simulink model "VariousSpeed2018_14dof_ypredictor_sc"  (R2017a)
settings: Solver=ode4  StartTime=0.0  StopTime=70  FixedStep=dt  RelTol=1e-3
values from neighbouring files (symbols this model uses):
  g_motor_eff = 1    [VESIM_init.m]
  gr_motor = 0    [VESIM_init.m]
undefined symbols (not defined in the file or in its folder): A_mc, brake_Pw, brake_V, C_q, diff_efficiency, diff_wRatio, dt, engine_inertia, error_lookuptable, F_cf, F_cs, fmin_mg, fmin_mg_na, J_cal, K_vb, Kp_rpm, mdot_fuel, model_lookuptable, no_cyl, P_0, P_gain, rpm0_c, rpm2rads, rpm_e, rpm_hi_idle, rpm_idle, rpm_max_c, rpm_rated, Standard_Devices, Ti_rpm, torque_engine, trq_scale, Tt_rpm, UDP_Protocol, vdes, Xobs, Yobs
libraries: simulink x10, vrlib x3, sldrtlib x3, SimulinkExecutionControl x1
(part 1 of 2)
settings Model: SimulationMode=accelerator  Creator=wenyifan  LastModifiedBy=Chen Li
settings SolverCC: AlgebraicLoopSolver=LineSearch
settings DataIOCC: LimitDataPoints=on  SaveFormat=Array
settings OptimizationCC: BlockReduction=off  BooleanDataType=off  LifeSpan=inf
settings DebuggingCC: SaveWithParameterizedLinksMsg=none  UnderspecifiedInitializationDetection=Classic  MergeDetectMultiDrivingBlocksExec=none  SignalResolutionControl=TryResolveAllWithWarning  AllowSymbolicDim=off  SFUnexpectedBacktrackingDiag=warning  SFNoUnconditionalDefaultTransitionDiag=warning  SFExecutionAtInitializationDiag=none
settings HardwareCC: TargetBitPerLong=64  TargetBitPerPointer=64  TargetIntDivRoundTo=Zero  TargetEndianess=LittleEndian  TargetWordSize=64  TargetHWDeviceType=Intel->x86-64
settings ModelReferenceCC: PropagateSignalLabelsOutOfModel=off
settings SFSimCC: MATLABDynamicMemAlloc=off
settings RTWCC: SystemTargetFile=sldrtert.tlc  TemplateMakefile=sldrtert.tmf  Description=Simulink Desktop Real-Time (ERT)  RTWCompilerOptimization=on
settings CodeAppCC: MaxIdLength=95
settings SimulinkDesktopRealTimeERTCC: TargetFcnLib=ansi_tfl_table_tmw.mat  TargetLibSuffix=_sldrt.lib  TargetPreCompLibLocation=E:\Matlab_2019a\toolbox\sldrt\lib\win64  GenFloatMathFcnCalls=NOT IN USE  TargetLangStandard=C89/C90 (ANSI)  CodeReplacementLibrary=None  UtilityFuncGeneration=Auto  MultiwordTypeDef=System defined  MultiwordLength=2048  GenerateFullHeader=on  InferredTypesCompatibility=off  GenerateSampleERTMain=off  GenerateTestInterfaces=off  ModelReferenceCompliant=on  ParMdlRefBuildCompliant=off  CompOptLevelCompliant=on  ConcurrentExecutionCompliant=off  IncludeMdlTerminateFcn=on  GeneratePreprocessorConditionals=Use local settings  CombineOutputUpdateFcns=off  CombineSignalStateStructs=off  SuppressErrorStatus=off  IncludeFileDelimiter=Auto  ERTCustomFileBanners=off  SupportAbsoluteTime=on  LogVarNameModifier=rt_  MatFileLogging=off  MultiInstanceERTCode=off  CodeInterfacePackaging=Nonreusable function  SupportNonFinite=on  SupportComplex=on  PurelyIntegerCode=off  SupportContinuousTime=on  SupportNonInlinedSFcns=on  RemoveDisableFunc=off  RemoveResetFunc=on  SupportVariableSizeSignals=off  ParenthesesLevel=Nominal  CastingMode=Nominal  MATLABClassNameForMDSCustomization=Simulink.SoftwareTarget.TargetSpecificTriggerConfigurationBase  ModelStepFunctionPrototypeControlCompliant=off  CPPClassGenCompliant=off  AutosarCompliant=off  MDXCompliant=off  GRTInterface=off  GenerateAllocFcn=off  UseToolchainInfoCompliant=off  GenerateSharedConstants=on  CoderGroups=[]  AccessMethods=[]  LookupTableObjectStructAxisOrder=1,2,3,4,...  GenerateASAP2=off  InlinedParameterPlacement=Hierarchical  TargetOS=BareBoardExample  MultiInstanceErrorCode=Error  RootIOFormat=Individual arguments  RTWCAPISignals=off  RTWCAPIParams=off  RTWCAPIStates=off  RTWCAPIRootIO=off  ERTSrcFileBannerTemplate=ert_code_template.cgt  ERTHdrFileBannerTemplate=ert_code_template.cgt  ERTDataSrcFileTemplate=ert_code_template.cgt  ERTDataHdrFileTemplate=ert_code_template.cgt  ERTCustomFileTemplate=example_file_process.tlc  EnableDataOwnership=off  SignalDisplayLevel=10  ParamTuneLevel=10  GlobalDataDefinition=Auto  DataDefinitionFile=global.c  GlobalDataReference=Auto  ERTFilePackagingFormat=Modular  DataReferenceFile=global.h  PreserveExpressionOrder=off  PreserveIfCondition=off  ConvertIfToSwitch=off  PreserveExternInFcnDecls=on  SuppressUnreachableDefaultCases=off  EnableSignedLeftShifts=on  EnableSignedRightShifts=on  IndentStyle=K&R  IndentSize=2  EnableUserReplacementTypes=off  MaxIdInt32=MAX_int32_T  MinIdInt32=MIN_int32_T  MaxIdUint32=MAX_uint32_T  MaxIdInt16=MAX_int16_T  MinIdInt16=MIN_int16_T  MaxIdUint16=MAX_uint16_T  MaxIdInt8=MAX_int8_T  MinIdInt8=MIN_int8_T  MaxIdUint8=MAX_uint8_T  BooleanTrueId=true  BooleanFalseId=false  MemSecPackage=--- None ---  MemSecDataConstants=Default  MemSecDataIO=Default  MemSecDataInternal=Default  MemSecDataParameters=Default  MemSecFuncInitTerm=Default  MemSecFuncExecute=Default  MemSecFuncSharedUtil=Default  GroupConstants=Default  GroupRootInputs=Default  GroupRootOutputs=Default  GroupInternal=Default  GroupParameters=Default  GroupDataTransfer=Default  GroupInstanceSpecificParameters=Default  GroupModelData=Default  CCListing=off  RebuildAll=off  ExtMode=on  ExtModeTransport=0  ExtModeStaticAlloc=off  ExtModeStaticAllocSize=1000000  ExtModeTesting=off  ExtModeMexFile=sldrtext  ExtModeIntrfLevel=Level1
settings ConfigComp: CovMetricSettings=dw  CovHtmlReporting=on  CovSaveCumulativeToWorkspaceVar=on  CovSaveSingleToWorkspaceVar=on  CovExternalEMLEnable=off  CovSFcnEnable=off

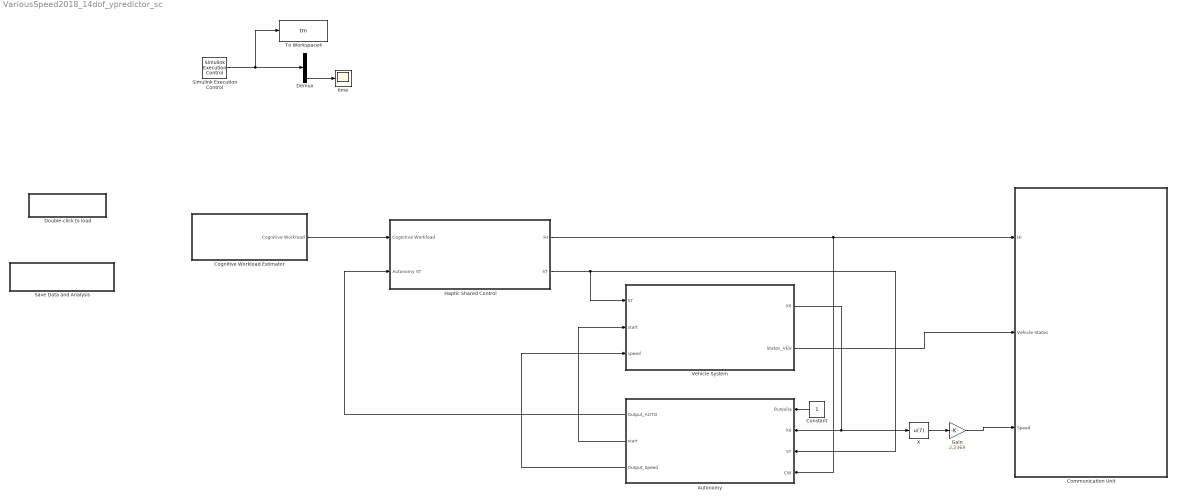
== system VariousSpeed2018_14dof_ypredictor_sc ==
  Autonomy : Subsystem
  Cognitive Workload Estimator : Subsystem
  Communication Unit : Subsystem
  Constant : Constant
  Demux : Demux  Outputs=3
  Double-click to load : Subsystem
      settings: OpenFcn=|
      | close all;
      | clear all;
      | clc;
      | 
      | env_init;
      | addpath(genpath(pwd))
      | 
      | 
      | VESIM_init;
      | VEHICLE14DoF_init;
      mask Help: This block runs/ndes_init.m file in the main directory
      mask Display: disp('Load Parameters')
  Gain : Gain  Gain=2.2369
  Haptic Shared Control : Subsystem
  Save Data and Analysis : Subsystem
      settings: OpenFcn=post_processing_analysis_pred_sc;
      mask Help: This block runs/ndes_init.m file in the main directory
      mask Display: disp('Save Data and Analysis')
  Simulink Execution Control : SimulinkExecutionControl/Simulink Execution Control  proc_pri=ABOVE_NORMAL_PRIORITY_CLASS  thread_pri=THREAD_PRIORITY_NORMAL  rt_sim=on  factor=1  ovrrun=Continue execution  Ts=dt
  To Workspace4 : ToWorkspace  VariableName=tm  SampleTime=-1
  Vehicle System : Subsystem
  X : Fcn  Expr=u(7)
  time : Scope
  wires:
  Simulink Execution Control/1 -> To Workspace4/1, Demux/1
  Vehicle System/1(X0) -> Autonomy/2(X0), X/1
  Constant/1 -> Autonomy/1(RunJulia)
  Haptic Shared Control/1(HI) -> Autonomy/4(CW), Communication Unit/1(HI)
  Demux/3 -> time/1
  Autonomy/3(Output_Speed) -> Vehicle System/3(speed)
  Gain/1 -> Communication Unit/3(Speed)
  Vehicle System/2(States_VEH) -> Communication Unit/2(Vehicle States)
  Autonomy/2(start) -> Vehicle System/2(start)
  X/1 -> Gain/1
  Autonomy/1(Output_AUTO) -> Haptic Shared Control/2(Autonomy ST)
  Cognitive Workload Estimator/1(Cognitive Workload) -> Haptic Shared Control/1(Cognitive Workload)
  Haptic Shared Control/2(ST) -> Vehicle System/1(ST), Autonomy/3(ST)

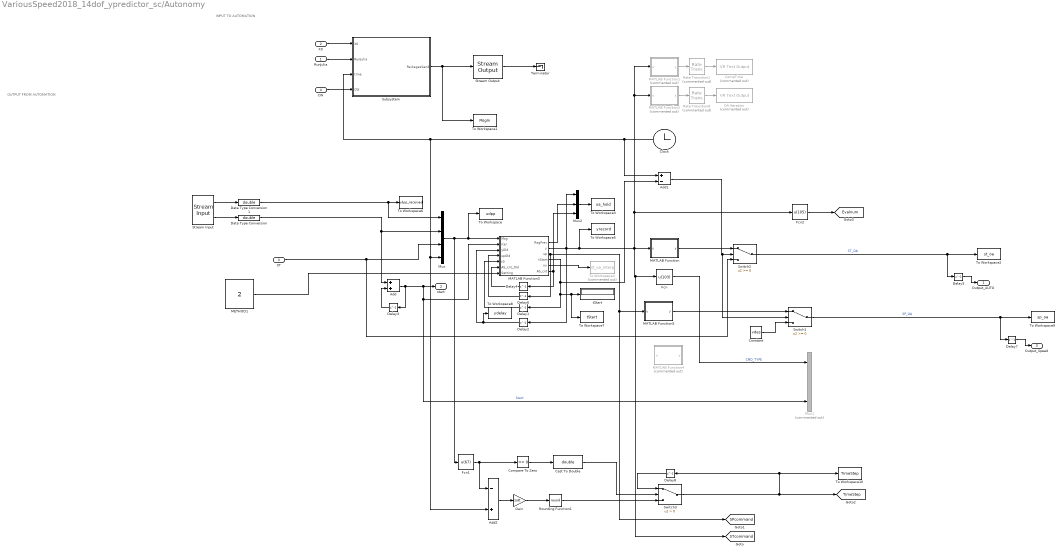
== system VariousSpeed2018_14dof_ypredictor_sc/Autonomy ==
  note: OUTPUT FROM AUTOMATION
  note: INPUT TO AUTOMATION
  RunJulia : Inport
  X0 : Inport  Port=2
  ST : Inport  Port=3
  CW : Inport  Port=4
  Add : Sum
  Add1 : Sum  Inputs=+-
  Add2 : Sum  Inputs=-+
  Cast To Double : DataTypeConversion  OutDataTypeStr=double
  Clock : Clock
      settings: Decimation=100
  CompTime : vrlib/VR Text Output  Commented=on  Ts=-1  ForceViewerOpen=off
      settings: SourceProductName=Simulink 3D Animation  SourceProductBaseCode=VR
  Compare To Zero : simulink/Logic and Bit Operations/Compare To Zero  relop===  OutDataTypeStr=boolean
  Constant : Constant  Value=vdes
  Data Type Conversion : DataTypeConversion  OutDataTypeStr=double
  Data Type Conversion1 : DataTypeConversion  OutDataTypeStr=double
  Delay{1,3..5,7..8} (6 alike) : Delay  DelayLength=1  InitialCondition=0  SampleTime=dt
  Delay2 : Delay  DelayLength=1  InitialCondition=zeros(110,1)  SampleTime=dt
  Delay6 : Delay  DelayLength=1  InitialCondition=zeros(110,1)  SampleTime=dt
  Fcn : Fcn  Expr=u(103)
  Fcn1 : Fcn  Expr=u(67)
  Fcn2 : Fcn  Expr=u(105)
  Gain : Gain  Gain=1/dt
  MATLAB Function : MATLAB Function  TreatAsAtomicUnit=on
  MATLAB Function1 : MATLAB Function  Commented=on  TreatAsAtomicUnit=on
  MATLAB Function2 : MATLAB Function  Commented=on  TreatAsAtomicUnit=on
  MATLAB Function3 : MATLAB Function  TreatAsAtomicUnit=on
  MATLAB Function4 : MATLAB Function  Commented=on  TreatAsAtomicUnit=on
  MATLAB Function5 : MATLAB Function  TreatAsAtomicUnit=on
  METHOD1 : Constant  Value=2
  Mux : Mux
  Mux1 : Mux  Commented=on  Inputs=3
  Mux2 : Mux  Inputs=3
  OA Iteration : vrlib/VR Text Output  Commented=on  Ts=-1  ForceViewerOpen=off
      settings: SourceProductName=Simulink 3D Animation  SourceProductBaseCode=VR
  Rate Transition1 : RateTransition  Commented=on
  Rate Transition8 : RateTransition  Commented=on
  Rounding Function1 : Rounding  Operator=round
  Stream Input : sldrtlib/Stream Input  SampleTime=0.01  MaxMissedTicks=Inf  ShowMissedTicks=off  YieldWhenWaiting=off  DrvName=Standard_Devices/UDP_Protocol  DrvAddress=36881  DrvOptions=[0 12000 51 53 46 51 46 57 57 46 49 57 53 0 0 0 0 0 0 0 0 0 0 0 0 0 0 0 0 0 0 0 0 0 0 0 0 0 0 0 0 0 0 0 0 0 0 0 0 0 0 0 0 0 0 0 0 0 0 0 0 0 0 0 0 0 0 0 0 0 0 0 0 0 0 0 0 0 0 0 0 0 0 0 0 0 0 0 0 0 0 0 0 0 0 0 0 0 0 0 0 0 0 0 0 0 0 0 0 0 0 0 0 0 0 0 0 0 0 0 0 0 0 0 0 0 0 0 0 0 0 0 0 0 0 0 0 0 0 0 0 0 0 0 0 0 0 0 0 0 0 0 0 0 0 0 0 0 0 0 0 0 0 0 0 0 0 0 0 0 0 0 0 0 0 0 0 0 0 0 0 0 0 0 0 0 0 0 0 0 0 0 0 0 0 0 0 0 0 0 0 0 0 0 0 0 0 0 0 0 0 0 0 0 0 0 0 0 0 0 0 0 0 0 0 0 0 0 0 0 0 0 0 0 0 0 0 0 0 0 0 0 0 0 0 0 0 0 0 0 0 0 0 0 0 0]  DataTypes={'68*double'}  FormatString='%f,%f,%f,%f,%f,%f,%f,%f,%f,%f,%f,%f,%f,%f,%f,%f,%f,%f,%f,%f,%f,%f,%f,%f,%f,%f,%f,%f,%f,%f,%f,%f,%f,%f,%f,%f,%f,%f,%f,%f,%f,%f,%f,%f,%f,%f,%f,%f,%f,%f,%f,%f,%f,%f,%f,%f,%f,%f,%f,%f,%f,%f,%f,%f,%f,%f,%f,%f'  Terminator={ '\r', '\n' }  ShowReady=on  ShowError=off
      settings: AttributesFormatString=UDP Protocol [36881]  SourceProductName=Simulink Desktop Real-Time  SourceProductBaseCode=WT
  Stream Output : sldrtlib/Stream Output  SampleTime=0.01  MaxMissedTicks=Inf  ShowMissedTicks=on  YieldWhenWaiting=off  DrvName=Standard_Devices/UDP_Protocol  DrvAddress=36864  DrvOptions=[0 36880 51 53 46 51 46 57 57 46 49 57 53 0 0 0 0 0 0 0 0 0 0 0 0 0 0 0 0 0 0 0 0 0 0 0 0 0 0 0 0 0 0 0 0 0 0 0 0 0 0 0 0 0 0 0 0 0 0 0 0 0 0 0 0 0 0 0 0 0 0 0 0 0 0 0 0 0 0 0 0 0 0 0 0 0 0 0 0 0 0 0 0 0 0 0 0 0 0 0 0 0 0 0 0 0 0 0 0 0 0 0 0 0 0 0 0 0 0 0 0 0 0 0 0 0 0 0 0 0 0 0 0 0 0 0 0 0 0 0 0 0 0 0 0 0 0 0 0 0 0 0 0 0 0 0 0 0 0 0 0 0 0 0 0 0 0 0 0 0 0 0 0 0 0 0 0 0 0 0 0 0 0 0 0 0 0 0 0 0 0 0 0 0 0 0 0 0 0 0 0 0 0 0 0 0 0 0 0 0 0 0 0 0 0 0 0 0 0 0 0 0 0 0 0 0 0 0 0 0 0 0 0 0 0 0 0 0 0 0 0 0 0 0 0 0 0 0 0 0 0 0 0 0 0 0]  PortSizes=[23]  FormatString='%f %f %f %f %f %f %f %f %f %f %f %f %f %f %f %f %f %f %f %f %f %f %f \n'  ShowReady=off  ShowError=off  InitialValue=[]  FinalValue=[]
      settings: AttributesFormatString=UDP Protocol [36864]  SourceProductName=Simulink Desktop Real-Time  SourceProductBaseCode=WT
  Subsystem : Subsystem
  Switch1 : Switch
  Switch2 : Switch
  Switch3 : Switch  Criteria=u2 > Threshold
  Terminator : Terminator
  To Workspace : ToWorkspace  VariableName=udpp  SampleTime=-1
      settings: Save2DSignal=2-D array (concatenate along first dimension)
  To Workspace1 : ToWorkspace  VariableName=MsgIn  SampleTime=-1
  To Workspace10 : ToWorkspace  VariableName=TimeStep  SampleTime=-1
  To Workspace2 : ToWorkspace  VariableName=st_oa  SampleTime=-1
  To Workspace3 : ToWorkspace  VariableName=oa_hold  SampleTime=-1
  To Workspace4 : ToWorkspace  Commented=on  VariableName=st_oa_interp  SampleTime=-1
  To Workspace5 : ToWorkspace  VariableName=yrecord  SampleTime=-1
      settings: Save2DSignal=2-D array (concatenate along first dimension)
  To Workspace6 : ToWorkspace  VariableName=udpp_received  SampleTime=-1
      settings: Save2DSignal=2-D array (concatenate along first dimension)
  To Workspace7 : ToWorkspace  VariableName=tStart  SampleTime=-1
  To Workspace8 : ToWorkspace  VariableName=ydelay  SampleTime=-1
      settings: Save2DSignal=2-D array (concatenate along first dimension)
  To Workspace9 : ToWorkspace  VariableName=sp_oa  SampleTime=-1
  tStart : Display
  Output_AUTO : Outport
  start : Outport  Port=2
  Output_Speed : Outport  Port=3
  tag scope: Evalnum=global, SPcommand=global, STcommand=global, TimeStep=global
  wires:
  Data Type Conversion1/1 -> Mux/1, To Workspace6/1
  MATLAB Function3/5(uu) -> To Workspace4/1
  MATLAB Function/1(y) -> Switch2/1
  Add1/1 -> Switch1/2, Switch2/2
  Add/1 -> Delay3/1, Mux1/3, MATLAB Function3/2(iter), start/1  "Start"
  Subsystem/1(PackagesSend) -> Stream Output/1, To Workspace1/1
  Rate Transition8/1 -> OA Iteration/1
  MATLAB Function3/6(AS_cnt) -> Mux2/3, Delay4/1
  Fcn/1 -> Mux1/1  "CMD_TYPE"
  MATLAB Function2/1(y) -> Rate Transition8/1
  Rate Transition1/1 -> CompTime/1
  MATLAB Function3/4(tStart) -> Add1/2, Delay1/1, To Workspace7/1, tStart/1
  Delay4/1 -> MATLAB Function3/6(AS_cnt_Old)
  RunJulia/1 -> Subsystem/2(RunJulia)
  MATLAB Function3/1(flagPrev) -> Mux2/2
  Delay1/1 -> MATLAB Function3/5(t0)
  Data Type Conversion/1 -> Add/1, Mux/2
  Mux2/1 -> To Workspace3/1
  METHOD1/1 -> MATLAB Function3/7(Setting)
  Delay3/1 -> Add/2
  Switch2/1 -> Delay5/1, To Workspace2/1  "ST_OA"
  X0/1 -> Subsystem/1(X0)
  MATLAB Function1/1(y) -> Rate Transition1/1
  Delay2/1 -> To Workspace8/1, MATLAB Function3/3(yOld)
  Stream Output/1 -> Terminator/1
  ST/1 -> Switch2/3, Mux/3
  Stream Input/2 -> Data Type Conversion/1
  Stream Input/1 -> Data Type Conversion1/1
  Delay5/1 -> Output_AUTO/1
  CW/1 -> Subsystem/4(CW)
  Delay6/1 -> MATLAB Function3/4(spOld)
  MATLAB Function5/1(y) -> Switch1/1
  Constant/1 -> Switch1/3
  Switch1/1 -> Delay7/1, To Workspace9/1  "SP_OA"
  Delay7/1 -> Output_Speed/1
  Delay8/1 -> Switch3/1
  Add2/1 -> Gain/1
  MATLAB Function3/3(sp) -> MATLAB Function5/1(u), [SPcommand], Delay6/1
  Cast To Double/1 -> Switch3/2
  Compare To Zero/1 -> Cast To Double/1
  Clock/1 -> Subsystem/3(time), Add2/2, Mux/4, Add1/1
  Mux/1 -> Fcn1/1, To Workspace/1, MATLAB Function3/1(Msg)
  Fcn1/1 -> Compare To Zero/1, Add2/1
  MATLAB Function3/2(y) -> Delay2/1, To Workspace5/1, [STcommand], Fcn/1, MATLAB Function1/1(u), MATLAB Function2/1(u), Fcn2/1, MATLAB Function/1(u), Mux2/1
  Fcn2/1 -> [Evalnum]
  Switch3/1 -> [TimeStep], Delay8/1, To Workspace10/1
  Gain/1 -> Rounding Function1/1
  Rounding Function1/1 -> Switch3/3

== system VariousSpeed2018_14dof_ypredictor_sc/Cognitive Workload Estimator ==
  Clock : Clock  Commented=on
  Constant : Constant
  MATLAB Function : MATLAB Function  Commented=on  TreatAsAtomicUnit=on
  Cognitive Workload : Outport
  wires:
  Constant/1 -> Cognitive Workload/1
  Clock/1 -> MATLAB Function/1(u)

== system VariousSpeed2018_14dof_ypredictor_sc/Communication Unit ==
  HI : Inport
  Vehicle States : Inport  Port=2
  Speed : Inport  Port=3
  Demux : Demux
  Mux : Mux  Inputs=6
  Stream Output : sldrtlib/Stream Output  SampleTime=0.01  MaxMissedTicks=Inf  ShowMissedTicks=on  YieldWhenWaiting=off  DrvName=Standard_Devices/UDP_Protocol  DrvAddress=10001  DrvOptions=[0 10002 51 53 46 51 46 50 57 46 51 53 0 0 0 0 0 0 0 0 0 0 0 0 0 0 0 0 0 0 0 0 0 0 0 0 0 0 0 0 0 0 0 0 0 0 0 0 0 0 0 0 0 0 0 0 0 0 0 0 0 0 0 0 0 0 0 0 0 0 0 0 0 0 0 0 0 0 0 0 0 0 0 0 0 0 0 0 0 0 0 0 0 0 0 0 0 0 0 0 0 0 0 0 0 0 0 0 0 0 0 0 0 0 0 0 0 0 0 0 0 0 0 0 0 0 0 0 0 0 0 0 0 0 0 0 0 0 0 0 0 0 0 0 0 0 0 0 0 0 0 0 0 0 0 0 0 0 0 0 0 0 0 0 0 0 0 0 0 0 0 0 0 0 0 0 0 0 0 0 0 0 0 0 0 0 0 0 0 0 0 0 0 0 0 0 0 0 0 0 0 0 0 0 0 0 0 0 0 0 0 0 0 0 0 0 0 0 0 0 0 0 0 0 0 0 0 0 0 0 0 0 0 0 0 0 0 0 0 0 0 0 0 0 0 0 0 0 0 0 0 0 0 0 0 0]  PortSizes=[6]  FormatString='%f %f %f %f %f %f\n'  ShowReady=off  ShowError=off  InitialValue=[]  FinalValue=[]
      settings: AttributesFormatString=UDP Protocol [10001]  SourceProductName=Simulink Desktop Real-Time  SourceProductBaseCode=WT
  Terminator : Terminator
  wires:
  Stream Output/1 -> Terminator/1
  Demux/4 -> Mux/4
  Vehicle States/1 -> Demux/1
  Demux/3 -> Mux/3
  Demux/2 -> Mux/2
  Demux/1 -> Mux/1
  HI/1 -> Mux/5
  Mux/1 -> Stream Output/1
  Speed/1 -> Mux/6

== system VariousSpeed2018_14dof_ypredictor_sc/Double-click to load ==
  note: double_click to load

== system VariousSpeed2018_14dof_ypredictor_sc/Haptic Shared Control ==
  Cognitive Workload : Inport
  Autonomy ST : Inport  Port=2
  Dead Zone : DeadZone  LowerValue=F_f_n  UpperValue=F_f_p  SaturateOnIntegerOverflow=on
  Delay1 : Delay  DelayLength=1
  Force Generator : Subsystem
  G29 Steering Wheel : Subsystem
  Subsystem2 : Subsystem
  Terminator : Terminator
  Terminator1 : Terminator
  To Workspace1 : ToWorkspace  VariableName=force_sc  SampleTime=-1
  To Workspace2 : ToWorkspace  VariableName=st_sc  SampleTime=-1
  To Workspace3 : ToWorkspace  VariableName=Predicted_ST  SampleTime=-1
  To Workspace4 : ToWorkspace  VariableName=HUM_INT  SampleTime=-1
  To Workspace5 : ToWorkspace  VariableName=tau_h  SampleTime=-1
  To Workspace6 : ToWorkspace  VariableName=force_sc_re  SampleTime=-1
  Trigger1 : Subsystem
  HI : Outport
  ST : Outport  Port=2
  wires:
  G29 Steering Wheel/3(BR) -> Terminator1/1
  G29 Steering Wheel/2(TH) -> Terminator/1
  Subsystem2/1(Predicted theta) -> To Workspace3/1
  Autonomy ST/1 -> Force Generator/2(Steering angle ref)
  Cognitive Workload/1 -> Force Generator/4(Cognitive Workload)
  Trigger1/1(Human's intervene Trigger) -> HI/1, Force Generator/6(human's intervention), To Workspace4/1
  Subsystem2/2(Predicted theta Error) -> Trigger1/1(Error)
  Subsystem2/3(Predicted Threshold) -> Trigger1/2(Threshold)
  Trigger1/2(PID reset) -> Force Generator/3(reset trigger)
  G29 Steering Wheel/1(ST) -> ST/1, To Workspace2/1, Subsystem2/2(Steering Angle), Force Generator/1(Steering angle)
  Force Generator/1(Force) -> Subsystem2/1(Force), Dead Zone/1, G29 Steering Wheel/1(Force), To Workspace1/1
  Dead Zone/1 -> Delay1/1
  Subsystem2/4(Predicted Human's Torque) -> To Workspace5/1, Force Generator/5(predicted human's torque)
  Delay1/1 -> To Workspace6/1

== system VariousSpeed2018_14dof_ypredictor_sc/Save Data and Analysis ==
  note: double_click to load

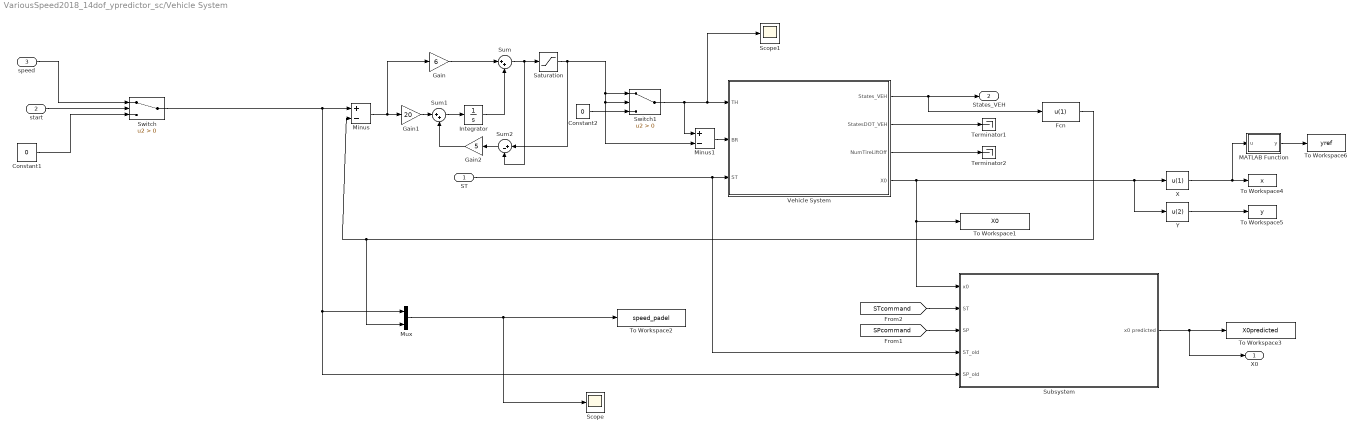
== system VariousSpeed2018_14dof_ypredictor_sc/Vehicle System ==
  ST : Inport
  start : Inport  Port=2
  speed : Inport  Port=3
  Constant1 : Constant  Value=0  SampleTime=dt
  Constant2 : Constant  Value=0  SampleTime=dt
  Fcn : Fcn  Expr=u(1)
  Gain : Gain  Gain=6
  Gain1 : Gain  Gain=20
  Gain2 : Gain  Gain=5
  Integrator : Integrator
  MATLAB Function : MATLAB Function  TreatAsAtomicUnit=on
  Minus : Sum  Inputs=+-
  Minus1 : Sum  Inputs=+-
  Mux : Mux  Inputs=2
  Saturation : Saturate  UpperLimit=1  LowerLimit=-1
  Scope : Scope
  Scope1 : Scope
  Subsystem : Subsystem
  Sum : Sum  Inputs=|++
  Sum1 : Sum  Inputs=|++
  Sum2 : Sum  Inputs=|+-
  Switch : Switch  Criteria=u2 > Threshold
  Switch1 : Switch  Criteria=u2 > Threshold
  Terminator1 : Terminator
  Terminator2 : Terminator
  To Workspace1 : ToWorkspace  VariableName=X0  SampleTime=-1
  To Workspace2 : ToWorkspace  VariableName=speed_padel  SampleTime=-1
  To Workspace3 : ToWorkspace  VariableName=X0predicted  SampleTime=-1
  To Workspace4 : ToWorkspace  VariableName=x  SampleTime=-1
  To Workspace5 : ToWorkspace  VariableName=y  SampleTime=-1
  To Workspace6 : ToWorkspace  VariableName=yref  SampleTime=-1
  Vehicle System : Subsystem
  X : Fcn  Expr=u(1)
  Y : Fcn  Expr=u(2)
  X0 : Outport
  States_VEH : Outport  Port=2
  wires:
  ST/1 -> Subsystem/4(ST_old), Vehicle System/3(ST)
  Vehicle System/1(States_VEH) -> Fcn/1, States_VEH/1
  Vehicle System/2(StatesDOT_VEH) -> Terminator1/1
  Vehicle System/3(NumTireLiftOff) -> Terminator2/1
  Fcn/1 -> Mux/2, Minus/2
  Minus/1 -> Gain1/1, Gain/1
  Gain/1 -> Sum/1
  Gain1/1 -> Sum1/1
  Sum1/1 -> Integrator/1
  Integrator/1 -> Sum/2
  Gain2/1 -> Sum1/2
  Sum2/1 -> Gain2/1
  Sum/1 -> Saturation/1, Sum2/2
  Saturation/1 -> Minus1/2, Switch1/2, Switch1/1, Sum2/1
  Switch1/1 -> Scope1/1, Vehicle System/1(TH), Minus1/1
  Constant2/1 -> Switch1/3
  Minus1/1 -> Vehicle System/2(BR)
  speed/1 -> Switch/1
  Constant1/1 -> Switch/3
  start/1 -> Switch/2
  Mux/1 -> Scope/1, To Workspace2/1
  Switch/1 -> Subsystem/5(SP_old), Mux/1, Minus/1
  [STcommand] -> Subsystem/2(ST)
  [SPcommand] -> Subsystem/3(SP)
  Subsystem/1(x0 predicted) -> X0/1, To Workspace3/1
  X/1 -> MATLAB Function/1(u), To Workspace4/1
  MATLAB Function/1(y) -> To Workspace6/1
  Y/1 -> To Workspace5/1
  Vehicle System/4(X0) -> Y/1, X/1, To Workspace1/1, Subsystem/1(x0)

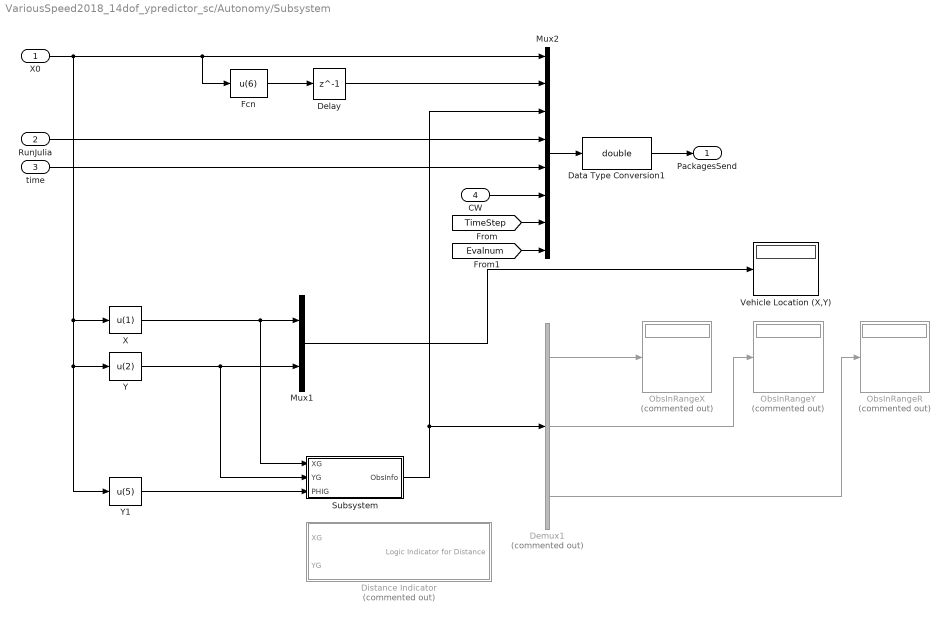
== system VariousSpeed2018_14dof_ypredictor_sc/Autonomy/Subsystem ==
  X0 : Inport
  RunJulia : Inport  Port=2
  time : Inport  Port=3
  CW : Inport  Port=4
  Data Type Conversion1 : DataTypeConversion  OutDataTypeStr=double
  Delay : Delay  DelayLength=1  InitialCondition=0  SampleTime=dt
  Demux1 : Demux  Commented=on  Outputs=[3 3 3]
  Distance Indicator : Subsystem  Commented=on
  Fcn : Fcn  Expr=u(6)
  Mux1 : Mux  Inputs=2
  Mux2 : Mux  Inputs=8
  ObsInRangeR : Display  Commented=on
  ObsInRangeX : Display  Commented=on
  ObsInRangeY : Display  Commented=on
  Subsystem : Subsystem
  Vehicle Location (X,Y) : Display
  X : Fcn  Expr=u(1)
  Y : Fcn  Expr=u(2)
  Y1 : Fcn  Expr=u(5)
  PackagesSend : Outport
  wires:
  Data Type Conversion1/1 -> PackagesSend/1
  Mux2/1 -> Data Type Conversion1/1
  X0/1 -> Y1/1, Y/1, X/1, Fcn/1, Mux2/1
  Y/1 -> Subsystem/2(YG), Mux1/2
  Subsystem/1(ObsInfo) -> Mux2/3, Demux1/1
  Mux1/1 -> Vehicle Location (X,Y)/1
  Demux1/1 -> ObsInRangeX/1
  Demux1/2 -> ObsInRangeY/1
  Demux1/3 -> ObsInRangeR/1
  time/1 -> Mux2/5
  RunJulia/1 -> Mux2/4
  Delay/1 -> Mux2/2
  Fcn/1 -> Delay/1
  Y1/1 -> Subsystem/3(PHIG)
  X/1 -> Subsystem/1(XG), Mux1/1
  CW/1 -> Mux2/6
  [TimeStep] -> Mux2/7
  [Evalnum] -> Mux2/8

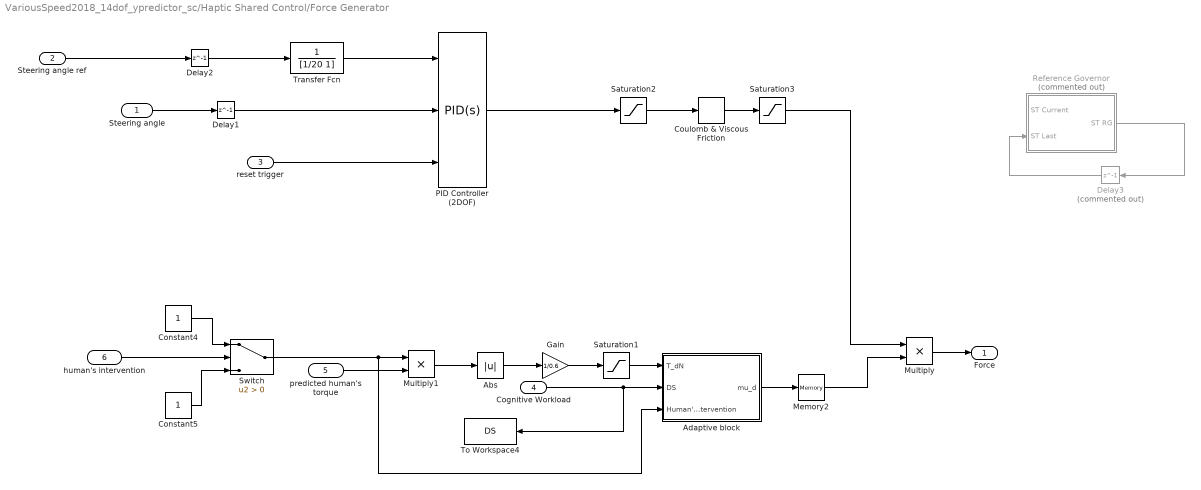
== system VariousSpeed2018_14dof_ypredictor_sc/Haptic Shared Control/Force Generator ==
  Steering angle : Inport
  Steering angle ref : Inport  Port=2
  reset trigger : Inport  Port=3
  Cognitive Workload : Inport  Port=4
  predicted human's torque : Inport  Port=5
  human's intervention : Inport  Port=6
  Abs : Abs
  Adaptive block : Subsystem
  Constant4 : Constant
  Constant5 : Constant
  Coulomb & Viscous Friction : simulink/Discontinuities/Coulomb & Viscous Friction  offset=0.12  gain=1
      settings: SourceProductName=Simulink
  Delay1 : Delay  DelayLength=1
  Delay2 : Delay  DelayLength=1
  Delay3 : Delay  Commented=on  DelayLength=1
  Gain : Gain  Gain=1/0.6
  Memory2 : Memory
  Multiply : Product
  Multiply1 : Product
  PID Controller (2DOF) : simulink/Continuous/PID Controller (2DOF)  Controller=PID  Form=Parallel  TimeDomain=Continuous-time  SampleTime=-1  IntegratorMethod=Forward Euler  FilterMethod=Forward Euler  ControllerParametersSource=internal  P=20  I=10  D=0.75  UseFilter=on  N=100  b=1  c=1  ZeroCross=off  InitialConditionSource=internal  InitialConditionForIntegrator=0  InitialConditionForFilter=0  DifferentiatorICPrevScaledInput=0  ExternalReset=rising  TrackingMode=off  Kt=1  LimitOutput=off  UpperSaturationLimit=inf  LowerSaturationLimit=-inf  LinearizeAsGain=on  AntiWindupMode=none  Kb=1  POutMin=[]  POutMax=[]  IOutMin=[]  IOutMax=[]  DOutMin=[]  DOutMax=[]  NOutMin=[]  NOutMax=[]  bOutMin=[]  bOutMax=[]  cOutMin=[]  cOutMax=[]  SumOutMin=[]  SumOutMax=[]  SaturationOutMin=[]  SaturationOutMax=[]  PParamMin=[]  PParamMax=[]  IParamMin=[]  IParamMax=[]  DParamMin=[]  DParamMax=[]  NParamMin=[]  NParamMax=[]  bParamMin=[]  bParamMax=[]  cParamMin=[]  cParamMax=[]  KbParamMin=[]  KbParamMax=[]  KtParamMin=[]  KtParamMax=[]  KbOutMin=[]  KbOutMax=[]  KtOutMin=[]  KtOutMax=[]  IntegratorOutMin=[]  IntegratorOutMax=[]  FilterOutMin=[]  FilterOutMax=[]  SumI1OutMin=[]  SumI1OutMax=[]  SumI2OutMin=[]  SumI2OutMax=[]  SumI3OutMin=[]  SumI3OutMax=[]  SumDOutMin=[]  SumDOutMax=[]  Sum1OutMin=[]  Sum1OutMax=[]  Sum2OutMin=[]  Sum2OutMax=[]  Sum3OutMin=[]  Sum3OutMax=[]  DifferentiatorOutMin=[]  DifferentiatorOutMax=[]  IntegratorContinuousStateAttributes=''  IntegratorStateMustResolveToSignalObject=off  IntegratorRTWStateStorageClass=Auto  FilterContinuousStateAttributes=''  FilterStateMustResolveToSignalObject=off  FilterRTWStateStorageClass=Auto
  Reference Governor : Subsystem  Commented=on
  Saturation1 : Saturate  UpperLimit=1  LowerLimit=0
  Saturation2 : Saturate  UpperLimit=0.59  LowerLimit=-0.59
  Saturation3 : Saturate  UpperLimit=0.59  LowerLimit=-0.59
  Switch : Switch  Criteria=u2 > Threshold
  To Workspace4 : ToWorkspace  VariableName=DS  SampleTime=-1
  Transfer Fcn : TransferFcn  Denominator=[1/20 1]
  Force : Outport
  wires:
  Steering angle/1 -> Delay1/1
  Delay1/1 -> PID Controller (2DOF)/2
  Saturation2/1 -> Coulomb & Viscous Friction/1
  PID Controller (2DOF)/1 -> Saturation2/1
  Coulomb & Viscous Friction/1 -> Saturation3/1
  Steering angle ref/1 -> Delay2/1
  Saturation3/1 -> Multiply/1
  Multiply/1 -> Force/1
  Adaptive block/1(mu_d) -> Memory2/1
  Cognitive Workload/1 -> To Workspace4/1, Adaptive block/2(DS)
  Memory2/1 -> Multiply/2
  Gain/1 -> Saturation1/1
  Abs/1 -> Gain/1
  Saturation1/1 -> Adaptive block/1(T_dN)
  predicted human's torque/1 -> Multiply1/2
  Switch/1 -> Adaptive block/3(Human's intervention), Multiply1/1
  Multiply1/1 -> Abs/1
  reset trigger/1 -> PID Controller (2DOF)/3
  Reference Governor/1(ST RG) -> Delay3/1
  Delay3/1 -> Reference Governor/2(ST Last)
  Delay2/1 -> Transfer Fcn/1
  Transfer Fcn/1 -> PID Controller (2DOF)/1
  Constant4/1 -> Switch/1
  Constant5/1 -> Switch/3
  human's intervention/1 -> Switch/2

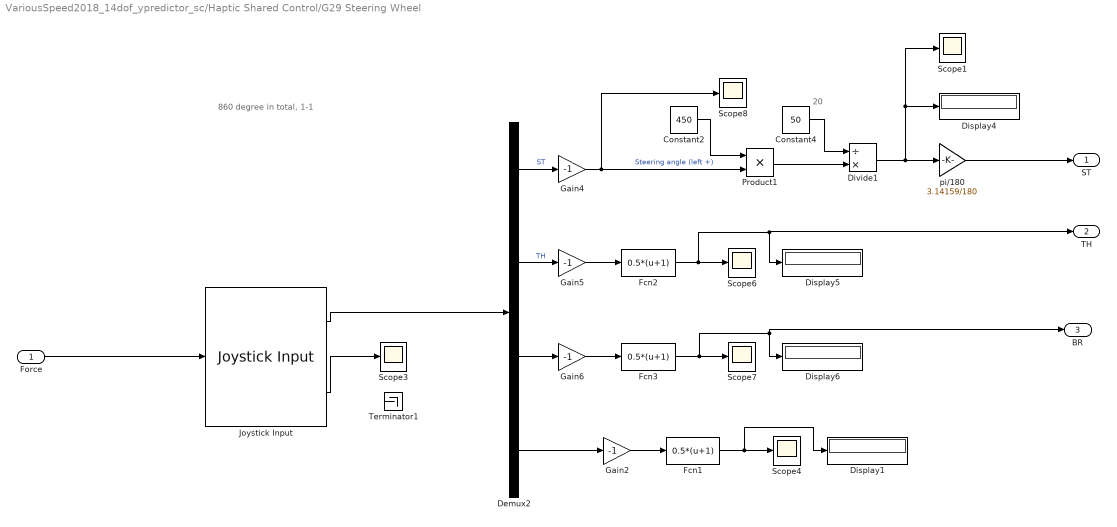
== system VariousSpeed2018_14dof_ypredictor_sc/Haptic Shared Control/G29 Steering Wheel ==
  note: 860 degree in total, 1-1
  note: 20
  Force : Inport
  Constant2 : Constant  Value=450
  Constant4 : Constant  Value=50
  Demux2 : Demux  Outputs=[1 1 1 1]
  Display{1,4..6} (4 alike) : Display
  Divide1 : Product  Inputs=/*
  Fcn1 : Fcn  Expr=0.5*(u+1)
  Fcn2 : Fcn  Expr=0.5*(u+1)
  Fcn3 : Fcn  Expr=0.5*(u+1)
  Gain{2,4..6} (4 alike) : Gain  Gain=-1
  Joystick Input : vrlib/Joystick Input  joyid=1  adjustports=on  forcefeed=on
      settings: SourceProductBaseCode=VR
  Product1 : Product
  Scope{1,3..4,6..8} (6 alike) : Scope
  Terminator1 : Terminator
  pi/180 : Gain  Gain=3.14159/180
  ST : Outport
  TH : Outport  Port=2
  BR : Outport  Port=3
  wires:
  Joystick Input/2 -> Scope3/1
  ? -> Terminator1/1
  Force/1 -> Joystick Input/1
  Joystick Input/1 -> Demux2/1
  Divide1/1 -> Scope1/1, Display4/1, pi/180/1
  Demux2/1 -> Gain4/1  "ST"
  Product1/1 -> Divide1/2
  Gain4/1 -> Product1/2, Scope8/1  "Steering angle (left +)"
  Constant4/1 -> Divide1/1
  pi/180/1 -> ST/1
  Constant2/1 -> Product1/1
  Fcn2/1 -> TH/1, Display5/1, Scope6/1
  Gain5/1 -> Fcn2/1
  Demux2/2 -> Gain5/1  "TH"
  Demux2/3 -> Gain6/1
  Fcn3/1 -> BR/1, Display6/1, Scope7/1
  Gain6/1 -> Fcn3/1
  Demux2/4 -> Gain2/1
  Fcn1/1 -> Display1/1, Scope4/1
  Gain2/1 -> Fcn1/1

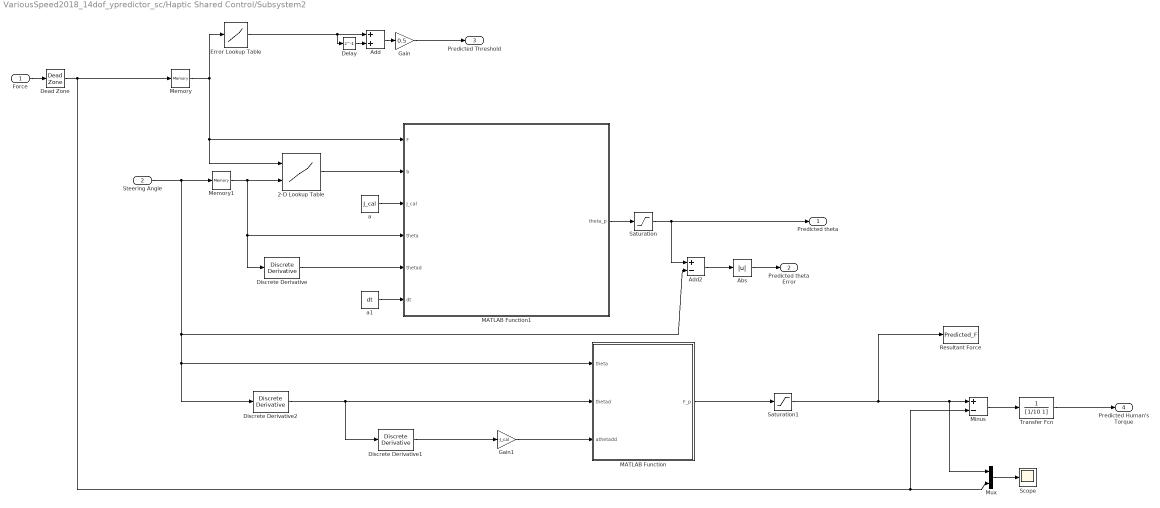
== system VariousSpeed2018_14dof_ypredictor_sc/Haptic Shared Control/Subsystem2 ==
  Force : Inport
  Steering Angle : Inport  Port=2
  2-D Lookup Table : Lookup_n-D  BreakpointsForDimension1=model_lookuptable.Breakpoints_row  BreakpointsForDimension2=model_lookuptable.Breakpoints_column  Table=model_lookuptable.Tabledata  InternalRulePriority=Speed  RndMeth=Simplest  InputSameDT=on
  Abs : Abs
  Add : Sum
  Add2 : Sum  Inputs=+-
  Dead Zone : DeadZone  LowerValue=F_f_n  UpperValue=F_f_p  SaturateOnIntegerOverflow=on
  Delay : Delay  DelayLength=1
  Discrete Derivative : simulink/Discrete/Discrete Derivative  gainval=1.0  ICPrevScaledInput=0.0  OutMin=[]  OutMax=[]  OutDataType=fixdt(1, 16)  OutScaling=2^-10  DoSatur=off
  Discrete Derivative1 : simulink/Discrete/Discrete Derivative  gainval=1.0  ICPrevScaledInput=0.0  OutMin=[]  OutMax=[]  OutDataType=fixdt(1, 16)  OutScaling=2^-10  DoSatur=off
  Discrete Derivative2 : simulink/Discrete/Discrete Derivative  gainval=1.0  ICPrevScaledInput=0.0  OutMin=[]  OutMax=[]  OutDataType=fixdt(1, 16)  OutScaling=2^-10  DoSatur=off
  Error Lookup Table : Lookup_n-D  NumberOfTableDimensions=1  BreakpointsForDimension1=error_lookuptable.Breakpoints  Table=error_lookuptable.Tabledata  InternalRulePriority=Speed  RndMeth=Simplest  InputSameDT=on
  Gain : Gain  Gain=0.5
  Gain1 : Gain  Gain=-J_cal
  MATLAB Function : MATLAB Function  TreatAsAtomicUnit=on
  MATLAB Function1 : MATLAB Function  TreatAsAtomicUnit=on
  Memory : Memory
  Memory1 : Memory
  Minus : Sum  Inputs=+-
  Mux : Mux  Inputs=2
  Resultant Force : ToWorkspace  VariableName=Predicted_F  SampleTime=-1
  Saturation : Saturate  UpperLimit=9/180*pi  LowerLimit=-9/180*pi
  Saturation1 : Saturate  UpperLimit=0.4386  LowerLimit=-0.4228
  Scope : Scope
  Transfer Fcn : TransferFcn  Denominator=[1/10 1]
  a : Constant  Value=J_cal
  a1 : Constant  Value=dt
  Predicted theta : Outport
  Predicted theta Error : Outport  Port=2
  Predicted Threshold : Outport  Port=3
  Predicted Human's Torque : Outport  Port=4
  wires:
  Discrete Derivative/1 -> MATLAB Function1/5(thetad)
  Saturation/1 -> Add2/1, Predicted theta/1
  Discrete Derivative1/1 -> Gain1/1
  Force/1 -> Dead Zone/1
  Gain1/1 -> MATLAB Function/3(athetadd)
  MATLAB Function/1(F_p) -> Saturation1/1
  Saturation1/1 -> Mux/1, Minus/1, Resultant Force/1
  Add2/1 -> Abs/1
  Abs/1 -> Predicted theta Error/1
  a/1 -> MATLAB Function1/3(J_cal)
  2-D Lookup Table/1 -> MATLAB Function1/2(b)
  MATLAB Function1/1(theta_p) -> Saturation/1
  a1/1 -> MATLAB Function1/6(dt)
  Steering Angle/1 -> Memory1/1, Add2/2, MATLAB Function/1(theta), Discrete Derivative2/1
  Memory/1 -> MATLAB Function1/1(F), 2-D Lookup Table/1, Error Lookup Table/1
  Memory1/1 -> Discrete Derivative/1, MATLAB Function1/4(theta), 2-D Lookup Table/2
  Discrete Derivative2/1 -> Discrete Derivative1/1, MATLAB Function/2(thetad)
  Delay/1 -> Add/2
  Error Lookup Table/1 -> Delay/1, Add/1
  Add/1 -> Gain/1
  Gain/1 -> Predicted Threshold/1
  Minus/1 -> Transfer Fcn/1
  Dead Zone/1 -> Minus/2, Mux/2, Memory/1
  Mux/1 -> Scope/1
  Transfer Fcn/1 -> Predicted Human's Torque/1

== system VariousSpeed2018_14dof_ypredictor_sc/Haptic Shared Control/Trigger1 ==
  Error : Inport
  Threshold : Inport  Port=2
  Compare To Constant : simulink/Logic and Bit Operations/Compare To Constant  relop===  const=0  OutDataTypeStr=boolean
  Compare To Constant1 : simulink/Logic and Bit Operations/Compare To Constant  relop===  const=1  OutDataTypeStr=boolean
  Delay1 : Delay  DelayLength=1  InitialCondition=zeros(1,10)
  Delay2 : Delay  DelayLength=1  InitialCondition=0
  Delay3 : Delay  DelayLength=1  InitialCondition=0
  Delay4 : Delay  DelayLength=1  InitialCondition=zeros(1,20)
  Logical Operator : Logic  AllPortsSameDT=off  OutDataTypeStr=boolean
  MATLAB Function : MATLAB Function  TreatAsAtomicUnit=on
  Terminator : Terminator
  Human's intervene Trigger : Outport
  PID reset : Outport  Port=2
  wires:
  MATLAB Function/3(tr_vect) -> Delay4/1
  Delay4/1 -> MATLAB Function/3(tr_vect_old)
  MATLAB Function/4(trigger) -> Delay2/1, Compare To Constant/1, Human's intervene Trigger/1
  MATLAB Function/1(vect) -> Delay1/1
  Delay1/1 -> MATLAB Function/2(vect_old)
  Threshold/1 -> MATLAB Function/4(threshold)
  Error/1 -> MATLAB Function/1(u)
  Logical Operator/1 -> Delay3/1
  Compare To Constant1/1 -> Logical Operator/2
  Compare To Constant/1 -> Logical Operator/1
  Delay2/1 -> Compare To Constant1/1
  MATLAB Function/2(flag) -> Terminator/1
  Delay3/1 -> PID reset/1

== system VariousSpeed2018_14dof_ypredictor_sc/Vehicle System/Subsystem ==
  x0 : Inport
  ST : Inport  Port=2
  SP : Inport  Port=3
  ST_old : Inport  Port=4
  SP_old : Inport  Port=5
  Constant : Constant  Value=dt
  Delay5 : Delay  DelayLength=1  InitialCondition=[zeros(103,1);1;zeros(6,1)]
  Delay6 : Delay  DelayLength=1  InitialCondition=[vdes*ones(103,1);1;zeros(6,1)]
  MATLAB Function2 : MATLAB Function  TreatAsAtomicUnit=on
  To Workspace2 : ToWorkspace  VariableName=STcommand  SampleTime=-1
  To Workspace3 : ToWorkspace  VariableName=SPcommand  SampleTime=-1
  To Workspace4 : ToWorkspace  VariableName=st_length  SampleTime=-1
  index : Fcn  Expr=u(104)
  x0 predicted : Outport
  wires:
  ST/1 -> Delay5/1
  x0/1 -> MATLAB Function2/1(X0)
  SP/1 -> Delay6/1
  Constant/1 -> MATLAB Function2/6(dt)
  index/1 -> MATLAB Function2/5(idx)
  [TimeStep] -> MATLAB Function2/4(time_step)
  MATLAB Function2/1(X0predicted) -> x0 predicted/1
  Delay5/1 -> To Workspace4/1, To Workspace2/1, index/1, MATLAB Function2/2(ST_length)
  Delay6/1 -> MATLAB Function2/3(SP_length), To Workspace3/1
  SP_old/1 -> MATLAB Function2/8(sp_old)
  ST_old/1 -> MATLAB Function2/7(st_old)

== system VariousSpeed2018_14dof_ypredictor_sc/Vehicle System/Vehicle System ==
  TH : Inport
  BR : Inport  Port=2
  ST : Inport  Port=3
  Derivative : Derivative
  Derivative1 : Derivative
  Hydraulic brake : Subsystem
  Mux1 : Mux  Inputs=8
  Mux2 : Mux
  Mux3 : Mux
  Powertrain1 : Subsystem
  Rate Transition : RateTransition
  Vehicle Model1 : Subsystem
  States_VEH : Outport
  StatesDOT_VEH : Outport  Port=2
  NumTireLiftOff : Outport  Port=3
  X0 : Outport  Port=4
  wires:
  Powertrain1/1(T shaft) -> Vehicle Model1/1(T_shaft)
  Vehicle Model1/1(w_shaft) -> Powertrain1/1(w shaft)
  Vehicle Model1/2(UG) -> Derivative/1, Mux1/7, Mux2/1
  Vehicle Model1/3(X) -> Mux1/1, Mux2/2
  Vehicle Model1/4(Y) -> Mux1/2, Mux2/3
  Vehicle Model1/5(PSI) -> Mux1/5, Derivative1/1, Mux2/4
  Vehicle Model1/8(YDOT) -> Mux3/3
  Vehicle Model1/7(XDOT) -> Mux3/2
  Mux3/1 -> StatesDOT_VEH/1
  Mux2/1 -> States_VEH/1
  Hydraulic brake/1(Brake torque) -> Vehicle Model1/2(Brake_cmd)
  Vehicle Model1/10(NumTireLiftOff) -> Rate Transition/1
  Rate Transition/1 -> NumTireLiftOff/1
  ST/1 -> Mux1/6, Vehicle Model1/3(Steering)
  Derivative/1 -> Mux3/1
  Derivative1/1 -> Mux3/4
  TH/1 -> Powertrain1/2(throttle)
  BR/1 -> Hydraulic brake/1(Brake command)
  Mux1/1 -> X0/1
  Vehicle Model1/9(PSIDOT) -> Mux1/4
  Vehicle Model1/6(UGDOT) -> Mux1/8
  Vehicle Model1/11(VG) -> Mux1/3

== system VariousSpeed2018_14dof_ypredictor_sc/Autonomy/Subsystem/Distance Indicator ==
  XG : Inport
  YG : Inport  Port=2
  Cast To Double : DataTypeConversion  OutDataTypeStr=double
  Compare To Constant : simulink/Logic and Bit Operations/Compare To Constant  relop=>=  const=0.5  OutDataTypeStr=boolean
  Delay1 : Delay  DelayLength=1  InitialCondition=0  SampleTime=dt
  Subsystem1 : Subsystem
  To Workspace4 : ToWorkspace  VariableName=distance_var  SampleTime=-1
  Logic Indicator for Distance : Outport
  wires:
  XG/1 -> Subsystem1/1(XG)
  Subsystem1/2(X_init_update) -> Delay1/1
  YG/1 -> Subsystem1/2(YG)
  Subsystem1/1(DisInfo) -> To Workspace4/1, Compare To Constant/1
  Delay1/1 -> Subsystem1/3(X_init)
  Compare To Constant/1 -> Cast To Double/1
  Cast To Double/1 -> Logic Indicator for Distance/1

== system VariousSpeed2018_14dof_ypredictor_sc/Autonomy/Subsystem/Subsystem ==
  XG : Inport
  YG : Inport  Port=2
  PHIG : Inport  Port=3
  Compare To Constant : simulink/Logic and Bit Operations/Compare To Constant  relop=<  const=900  OutDataTypeStr=boolean
  Data Type Conversion : DataTypeConversion  OutDataTypeStr=double
  Fcn : Fcn  Expr=u(1)
  MATLAB Function : MATLAB Function  TreatAsAtomicUnit=on
  Mux : Mux  Inputs=3
  ObsR : Constant  Value=[1 1 1]  SampleTime=dt
  Saturation : Saturate  UpperLimit=900  LowerLimit=0
  Saturation1 : Saturate  UpperLimit=900  LowerLimit=0
  Xobs : Constant  Value=Xobs  SampleTime=dt
  Yobs : Constant  Value=Yobs  SampleTime=dt
  vdes : Constant  Value=vdes  SampleTime=dt
  ObsInfo : Outport
  tag scope: Obsinfo=global
  wires:
  Xobs/1 -> MATLAB Function/4(Xobs)
  Yobs/1 -> MATLAB Function/5(Yobs)
  XG/1 -> MATLAB Function/1(XG)
  YG/1 -> MATLAB Function/2(YG)
  PHIG/1 -> MATLAB Function/3(PHIG)
  MATLAB Function/1(Xobs_pass) -> Saturation/1
  Saturation/1 -> Fcn/1, Mux/1
  Saturation1/1 -> Mux/2
  Mux/1 -> ObsInfo/1
  ObsR/1 -> Mux/3
  MATLAB Function/2(Yobs_pass) -> Saturation1/1
  vdes/1 -> MATLAB Function/6(vdes)
  Compare To Constant/1 -> Data Type Conversion/1
  Data Type Conversion/1 -> [Obsinfo]
  Fcn/1 -> Compare To Constant/1

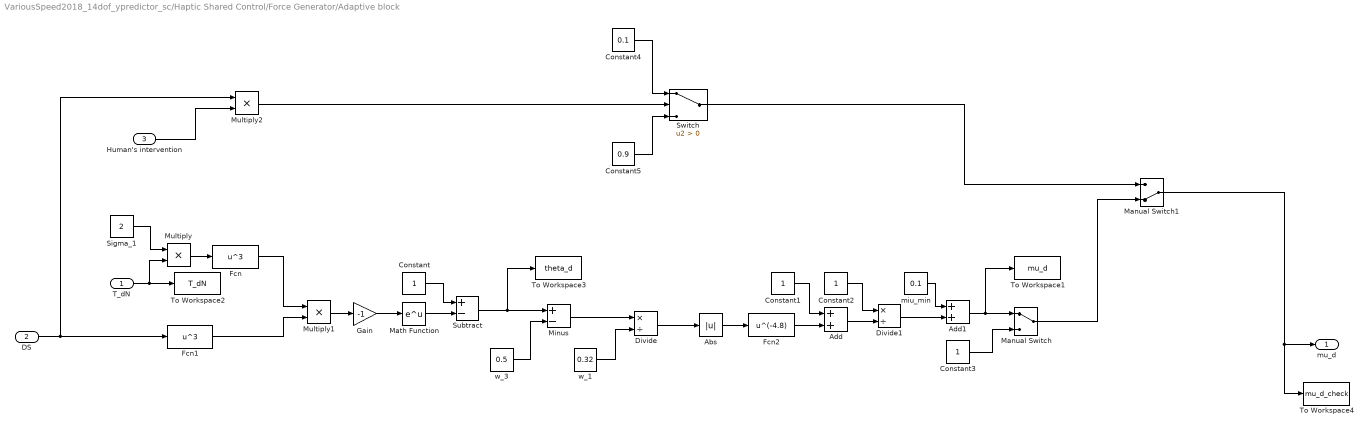
== system VariousSpeed2018_14dof_ypredictor_sc/Haptic Shared Control/Force Generator/Adaptive block ==
  T_dN : Inport
  DS : Inport  Port=2
  Human's intervention : Inport  Port=3
  Abs : Abs
  Add : Sum
  Add1 : Sum
  Constant{,1..3} (4 alike) : Constant
  Constant4 : Constant  Value=0.1
  Constant5 : Constant  Value=0.9
  Divide : Product  Inputs=*/
  Divide1 : Product  Inputs=*/
  Fcn : Fcn  Expr=u^3
  Fcn1 : Fcn  Expr=u^3
  Fcn2 : Fcn  Expr=u^(-4.8)
  Gain : Gain  Gain=-1
  Manual Switch : ManualSwitch
  Manual Switch1 : ManualSwitch  CurrentSetting=0
  Math Function : Math  SaturateOnIntegerOverflow=on
  Minus : Sum  Inputs=+-
  Multiply : Product
  Multiply1 : Product
  Multiply2 : Product
  Sigma_1 : Constant  Value=2
  Subtract : Sum  Inputs=+-
  Switch : Switch  Criteria=u2 > Threshold
  To Workspace1 : ToWorkspace  VariableName=mu_d  SampleTime=-1
  To Workspace2 : ToWorkspace  VariableName=T_dN  SampleTime=-1
  To Workspace3 : ToWorkspace  VariableName=theta_d  SampleTime=-1
  To Workspace4 : ToWorkspace  VariableName=mu_d_check  SampleTime=-1
  miu_min : Constant  Value=0.1
  w_1 : Constant  Value=0.32
  w_3 : Constant  Value=0.5
  mu_d : Outport
  wires:
  Sigma_1/1 -> Multiply/1
  T_dN/1 -> Multiply/2, To Workspace2/1
  Multiply/1 -> Fcn/1
  Fcn/1 -> Multiply1/1
  Fcn1/1 -> Multiply1/2
  Multiply1/1 -> Gain/1
  Gain/1 -> Math Function/1
  Math Function/1 -> Subtract/2
  Constant/1 -> Subtract/1
  Subtract/1 -> Minus/1, To Workspace3/1
  w_3/1 -> Minus/2
  Minus/1 -> Divide/1
  w_1/1 -> Divide/2
  Divide/1 -> Abs/1
  Abs/1 -> Fcn2/1
  Fcn2/1 -> Add/2
  Constant1/1 -> Add/1
  Add/1 -> Divide1/2
  Constant2/1 -> Divide1/1
  Divide1/1 -> Add1/2
  miu_min/1 -> Add1/1
  Add1/1 -> Manual Switch/1, To Workspace1/1
  Manual Switch1/1 -> To Workspace4/1, mu_d/1
  Constant3/1 -> Manual Switch/2
  Manual Switch/1 -> Manual Switch1/2
  DS/1 -> Multiply2/1, Fcn1/1
  Human's intervention/1 -> Multiply2/2
  Multiply2/1 -> Switch/2
  Constant4/1 -> Switch/1
  Constant5/1 -> Switch/3
  Switch/1 -> Manual Switch1/1

== system VariousSpeed2018_14dof_ypredictor_sc/Haptic Shared Control/Force Generator/Reference Governor ==
  ST Current : Inport
  ST Last : Inport  Port=2
  MATLAB Function : MATLAB Function  TreatAsAtomicUnit=on
  ST RG : Outport
  wires:
  ST Current/1 -> MATLAB Function/1(ST_C)
  ST Last/1 -> MATLAB Function/2(ST_L)
  MATLAB Function/1(ST_RG) -> ST RG/1

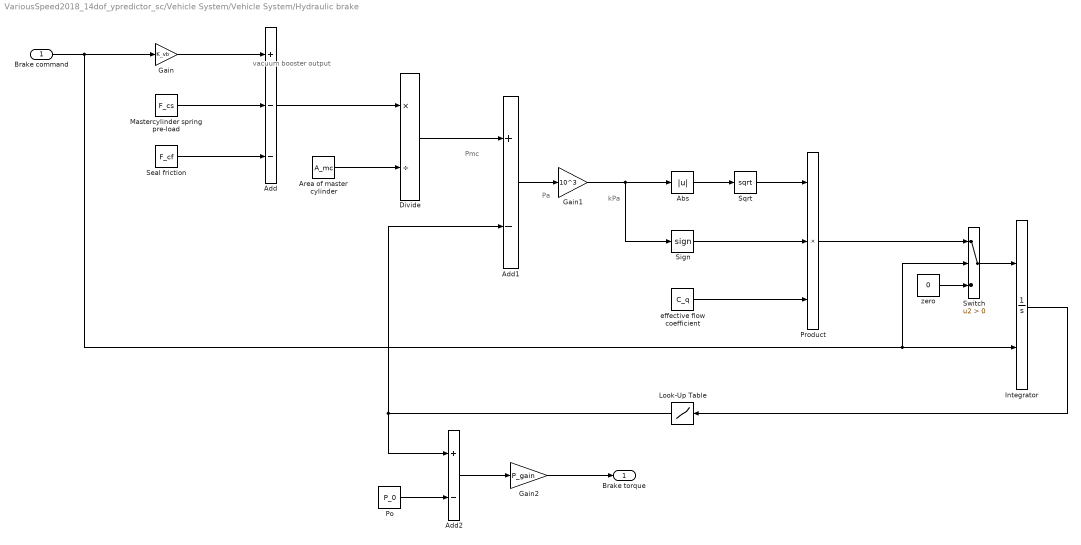
== system VariousSpeed2018_14dof_ypredictor_sc/Vehicle System/Vehicle System/Hydraulic brake ==
  note: kPa
  note: Pa
  note: Pmc
  note: vacuum booster output
  Brake command : Inport
  Abs : Abs
  Add : Sum  Inputs=+--
  Add1 : Sum  Inputs=+-
  Add2 : Sum  Inputs=+-
  Area of master cylinder : Constant  Value=A_mc
  Divide : Product  Inputs=*/
  Gain : Gain  Gain=K_vb
  Gain1 : Gain  Gain=10^3
  Gain2 : Gain  Gain=P_gain
  Integrator : Integrator  ExternalReset=either
  Look-Up Table : Lookup  InputValues=brake_V  Table=brake_Pw  SaturateOnIntegerOverflow=on
  Mastercylinder spring pre-load : Constant  Value=F_cs
  Po : Constant  Value=P_0
  Product : Product  Inputs=3
  Seal friction : Constant  Value=F_cf
  Sign : Signum
  Sqrt : Sqrt  SaturateOnIntegerOverflow=on
  Switch : Switch  Criteria=u2 > Threshold  SaturateOnIntegerOverflow=on  InputSameDT=on
  effective flow coefficient : Constant  Value=C_q
  zero : Constant  Value=0
  Brake torque : Outport
  wires:
  Brake command/1 -> Switch/2, Integrator/2, Gain/1
  Gain/1 -> Add/1
  Mastercylinder spring pre-load/1 -> Add/2
  Seal friction/1 -> Add/3
  Add/1 -> Divide/1
  Area of master cylinder/1 -> Divide/2
  Divide/1 -> Add1/1
  Add1/1 -> Gain1/1
  Abs/1 -> Sqrt/1
  Sqrt/1 -> Product/1
  Sign/1 -> Product/2
  effective flow coefficient/1 -> Product/3
  Gain1/1 -> Sign/1, Abs/1
  Look-Up Table/1 -> Add1/2, Add2/1
  Po/1 -> Add2/2
  Add2/1 -> Gain2/1
  Gain2/1 -> Brake torque/1
  Integrator/1 -> Look-Up Table/1
  Switch/1 -> Integrator/1
  Product/1 -> Switch/1
  zero/1 -> Switch/3

== system VariousSpeed2018_14dof_ypredictor_sc/Vehicle System/Vehicle System/Powertrain1 ==
  w shaft : Inport
  throttle : Inport  Port=2
  Constant : Constant  Value=0
  DIESEL ENGINE : Subsystem
  DRIVELINE : Subsystem
  Terminator1 : Terminator
  T shaft : Outport
  wires:
  throttle/1 -> DIESEL ENGINE/2(driver  demand), DRIVELINE/3(demand)
  w shaft/1 -> DRIVELINE/4(w shaft)
  DRIVELINE/2(T shaft) -> T shaft/1
  DRIVELINE/1(w pump) -> DIESEL ENGINE/1(engine speed)
  DIESEL ENGINE/1(engine torque) -> DRIVELINE/1("T eng ")
  Constant/1 -> DRIVELINE/2(T motor)
  DRIVELINE/3(w motor) -> Terminator1/1

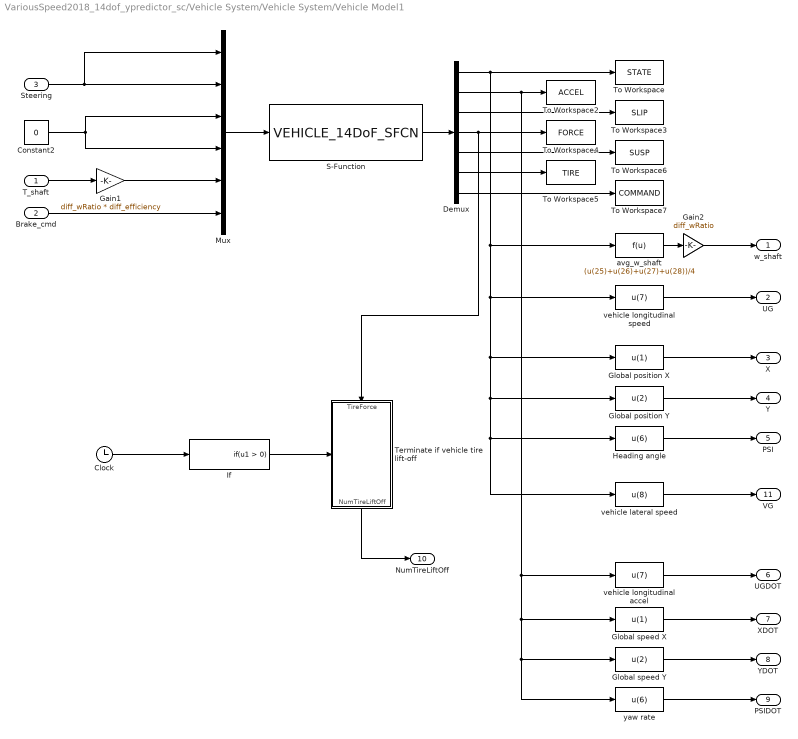
== system VariousSpeed2018_14dof_ypredictor_sc/Vehicle System/Vehicle System/Vehicle Model1 ==
  T_shaft : Inport
  Brake_cmd : Inport  Port=2
  Steering : Inport  Port=3
  Clock : Clock
  Constant2 : Constant  Value=0
  Demux : Demux  Outputs=[32,32,8,29,36,24,6]
  Gain1 : Gain  Gain=diff_wRatio * diff_efficiency
  Gain2 : Gain  Gain=diff_wRatio
  Global position X : Fcn  Expr=u(1)
  Global position Y : Fcn  Expr=u(2)
  Global speed X : Fcn  Expr=u(1)
  Global speed Y : Fcn  Expr=u(2)
  Heading angle : Fcn  Expr=u(6)
  If : If  ShowElse=off
  Mux : Mux  Inputs=6
  S-Function : S-Function  FunctionName=VEHICLE_14DoF_SFCN  SFunctionDeploymentMode=off  EnableBusSupport=off
  Terminate if vehicle tire lift-off : Subsystem  TreatAsAtomicUnit=on
  To Workspace : ToWorkspace  VariableName=STATE  SampleTime=-1
  To Workspace2 : ToWorkspace  VariableName=ACCEL  SampleTime=-1
  To Workspace3 : ToWorkspace  VariableName=SLIP  SampleTime=-1
  To Workspace4 : ToWorkspace  VariableName=FORCE  SampleTime=-1
  To Workspace5 : ToWorkspace  VariableName=TIRE  SampleTime=-1
  To Workspace6 : ToWorkspace  VariableName=SUSP  SampleTime=-1
  To Workspace7 : ToWorkspace  VariableName=COMMAND  SampleTime=-1
  avg_w_shaft : Fcn  Expr=(u(25)+u(26)+u(27)+u(28))/4
  vehicle lateral speed : Fcn  Expr=u(8)
  vehicle longitudinal accel : Fcn  Expr=u(7)
  vehicle longitudinal speed : Fcn  Expr=u(7)
  yaw rate : Fcn  Expr=u(6)
  w_shaft : Outport
  UG : Outport  Port=2
  X : Outport  Port=3
  Y : Outport  Port=4
  PSI : Outport  Port=5
  UGDOT : Outport  Port=6
  XDOT : Outport  Port=7
  YDOT : Outport  Port=8
  PSIDOT : Outport  Port=9
  NumTireLiftOff : Outport  Port=10
  VG : Outport  Port=11
  wires:
  Demux/3 -> To Workspace3/1
  Constant2/1 -> Mux/3, Mux/4
  Demux/5 -> To Workspace6/1
  Steering/1 -> Mux/1, Mux/2
  avg_w_shaft/1 -> Gain2/1
  T_shaft/1 -> Gain1/1
  Demux/7 -> To Workspace7/1
  Demux/1 -> To Workspace/1, vehicle lateral speed/1, Heading angle/1, Global position Y/1, Global position X/1, vehicle longitudinal speed/1, avg_w_shaft/1
  Mux/1 -> S-Function/1
  vehicle longitudinal speed/1 -> UG/1
  Demux/6 -> To Workspace5/1
  Brake_cmd/1 -> Mux/6
  S-Function/1 -> Demux/1
  Heading angle/1 -> PSI/1
  Gain2/1 -> w_shaft/1
  Gain1/1 -> Mux/5
  Global position X/1 -> X/1
  Global position Y/1 -> Y/1
  yaw rate/1 -> PSIDOT/1
  Demux/2 -> vehicle longitudinal accel/1, Global speed X/1, Global speed Y/1, yaw rate/1, To Workspace2/1
  vehicle longitudinal accel/1 -> UGDOT/1
  Global speed X/1 -> XDOT/1
  Global speed Y/1 -> YDOT/1
  Demux/4 -> Terminate if vehicle tire lift-off/1(TireForce), To Workspace4/1
  Clock/1 -> If/1
  If/1 -> Terminate if vehicle tire lift-off/Action
  Terminate if vehicle tire lift-off/1(NumTireLiftOff) -> NumTireLiftOff/1
  vehicle lateral speed/1 -> VG/1

== system VariousSpeed2018_14dof_ypredictor_sc/Autonomy/Subsystem/Distance Indicator/Subsystem1 ==
  XG : Inport
  YG : Inport  Port=2
  X_init : Inport  Port=3
  Constant : Constant  Value=0.01
  MATLAB Function : MATLAB Function  TreatAsAtomicUnit=on
  DisInfo : Outport
  X_init_update : Outport  Port=2
  wires:
  X_init/1 -> MATLAB Function/3(Xinit)
  YG/1 -> MATLAB Function/2(Yv)
  XG/1 -> MATLAB Function/1(Xv)
  Constant/1 -> MATLAB Function/4(alpha)
  MATLAB Function/1(Xinit_final) -> X_init_update/1
  MATLAB Function/2(distance) -> DisInfo/1

== system VariousSpeed2018_14dof_ypredictor_sc/Vehicle System/Vehicle System/Powertrain1/DIESEL ENGINE ==
  note: RPM
  note: If you are using MATLAB 6 or earlier,
      | double-click on this look-up table and
      | make sure the "Table data" entry is torque_engine
  engine speed : Inport
  driver  demand : Inport  Port=2
  Engine Map : Lookup2D  RowIndex=rpm_engine  ColumnIndex=mdot_fuel*1e3  Table=torque_engine  SaturateOnIntegerOverflow=on  InputSameDT=on
  Fuel controller/ Governor : Subsystem
  Gain : Gain  Gain=trq_scale  SaturateOnIntegerOverflow=on  OutDataTypeStr=Inherit: Same as input  ParamDataTypeStr=Inherit: Same as input
  Idle Controller : Subsystem
  Mux2 : Mux  Inputs=2
  To File1 : ToFile  Filename=Powertrain_data/engine_NO.mat  MatrixName=engine_out
  radpersec2rpm : Gain  Gain=1/rpm2rads
  engine torque : Outport
  wires:
  radpersec2rpm/1 -> Engine Map/1, Fuel controller/ Governor/2(rpm), Idle Controller/1(engine speed), Mux2/2
  engine speed/1 -> radpersec2rpm/1
  Fuel controller/ Governor/1(mdot_fuel) -> Engine Map/2
  Idle Controller/1(rack) -> Fuel controller/ Governor/1(Rack)
  Gain/1 -> engine torque/1, Mux2/1
  Mux2/1 -> To File1/1
  driver  demand/1 -> Idle Controller/2(driver command)
  Engine Map/1 -> Gain/1

== system VariousSpeed2018_14dof_ypredictor_sc/Vehicle System/Vehicle System/Powertrain1/DRIVELINE ==
  note: pump.e
  note: shaft.e
  note: T_motor.f
  note: w_Turbine_out
      | pump.e
      | w_ratio_disp
  note: shaft.e
      | T_turbine_out
  note: w_out_trans_out
  note: pump.e
      | trans_T_ratio_out
      | gear_out
  "T eng " : Inport
  T motor : Inport  Port=2
  demand : Inport  Port=3
  w shaft : Inport  Port=4
  Constant : Constant  Value=0
  Drivetrain1 : Subsystem  mask(20-sim 4.1 S-Function block){}
      mask help:
      | This block is generated by the 20-sim ANSI-C Code Generator.
      |
      | * look under the mask to get information on the ports
      | * press Help for more detailed information
      | * the parameters of this block are:
      mask Help:
      | This block is generated by the 20-sim ANSI-C Code Generator<br>
      | The block parameters are:<br><blockquote></blockquote>
      | Generated at:<br>
      | <blockquote><b>date:  </b>November 7, 2011<br>
      | <b>time:  </b>6:10:49 pm<br></blockquote>
      | From the following 20-sim model:<br>
      | <blockquote><b>submodel:  </b>Drivetrain<br>
      | <b>model:  </b>model-based internet integration - original drivetrain params<br>
      | <b>file:  </b>C:\Users\Tulga Ersal\Documents\U of M\Post Doc\Projects\Long-haul HIL integration\20-sim\integration models for 20Sim 4.0.1.5 and up\model-based internet integration - original drivetrain params.emx<br>
      | <b>experiment:  </b>C:\Users\Tulga Ersal\Documents\U of M\Post Doc\Projects\Long-haul HIL integration\20-sim\integration models for 20Sim 4.0.1.5 and up\model-based internet integration - original drivetrain params.emx<br></blockquote>
      | Using the following 20-sim license:<br>
      | <blockquote><b>user:  </b>The University of Michigan<br>
      | <b>from:  </b>Student License<br>
      | <b>build: </b>4.1.0.4<br></blockquote>
      mask Display: disp('Drivetrain')
  Mux1 : Mux  Inputs=3
  Mux2 : Mux  Inputs=2
  Mux3 : Mux  Inputs=3
  Terminator1 : Terminator
  To File1 : ToFile  Filename=Powertrain_data/Transmission_NO.mat  MatrixName=Transmission_out
  To File2 : ToFile  Filename=Powertrain_data/Prop_Diff_NO.mat  MatrixName=Prop_Diff_out
  To File3 : ToFile  Filename=Powertrain_data/ShiftLogic_NO.mat  MatrixName=ShiftLogic_out
  ToFile : ToFile  Filename=Powertrain_data/TC_NO.mat  MatrixName=TC_out
  engine dynamics (flywheel inertia only) : Subsystem
  gear ratio1 : Gain  Gain=gr_motor  SaturateOnIntegerOverflow=on  OutDataTypeStr=Inherit: Same as input  ParamDataTypeStr=Inherit: Same as input
  gear eff : Gain  Gain=g_motor_eff  SaturateOnIntegerOverflow=on  OutDataTypeStr=Inherit: Same as input  ParamDataTypeStr=Inherit: Same as input
  w pump : Outport  InitialOutput=0
  T shaft : Outport  Port=2  InitialOutput=0
  w motor : Outport  Port=3  InitialOutput=0
  wires:
  "T eng "/1 -> engine dynamics (flywheel inertia only)/1(brake torque)
  engine dynamics (flywheel inertia only)/1(rad/s) -> Drivetrain1/2(pump_f), w pump/1
  demand/1 -> Drivetrain1/1(demand)
  w shaft/1 -> Drivetrain1/3(shaft_f)
  T motor/1 -> gear eff/1
  gear eff/1 -> gear ratio1/1
  Constant/1 -> w motor/1
  Mux1/1 -> ToFile/1
  Mux2/1 -> To File1/1
  Mux3/1 -> To File3/1
  gear ratio1/1 -> Terminator1/1
  Drivetrain1/4(shaft_e) -> T shaft/1, Mux2/1
  Drivetrain1/3(pump_e) -> Mux3/1, Mux1/2, engine dynamics (flywheel inertia only)/2(Load Torque)
  Drivetrain1/13(w_Turbine_out) -> Mux1/1
  Drivetrain1/12(w_ratio_disp) -> Mux1/3
  Drivetrain1/10(T_turbine_out) -> Mux2/2
  Drivetrain1/11(w_out_trans_out) -> To File2/1
  Drivetrain1/9(trans_T_ratio_out) -> Mux3/2
  Drivetrain1/1(gear_out) -> Mux3/3
